simulink model "Periptwsi_2"  (R2020a)
settings: Solver=VariableStepAuto  StartTime=0.0  StopTime=20.0  RelTol=1e-3
undefined symbols (not defined in the file or in its folder): sigbuilder_block
libraries: fuzblock x2
settings Model: Creator=Vasilis Kyrgyrides  LastModifiedBy=Vasilis Kyrgyrides

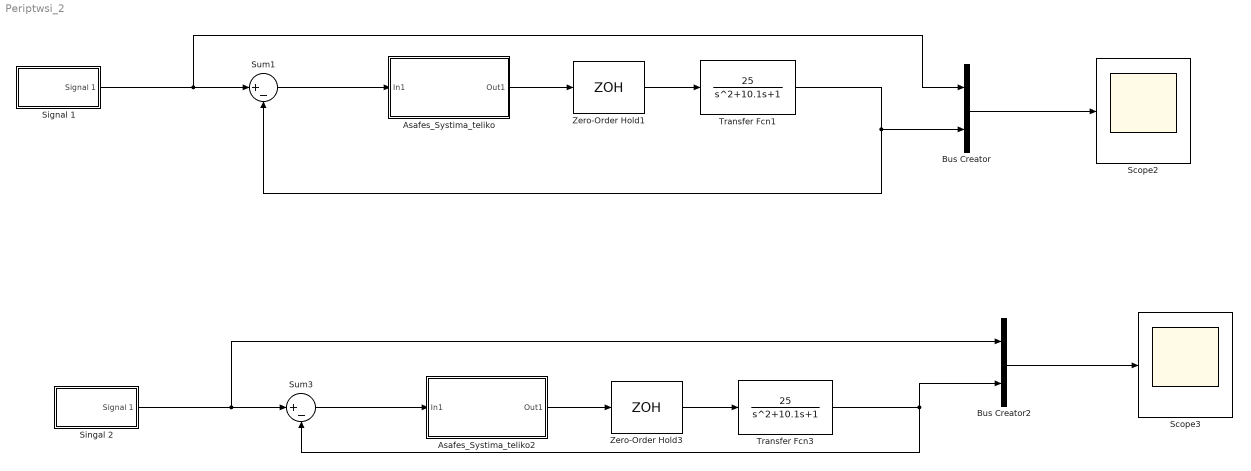
== system Periptwsi_2 ==
  Asafes_Systima_teliko : Subsystem
  Asafes_Systima_teliko2 : Subsystem
  Bus Creator : BusCreator  Inputs=2
  Bus Creator2 : BusCreator  Inputs=2
  Scope2 : Scope
  Scope3 : Scope
  Signal 1 : Subsystem  Tag=STV Subsys  LoadFcn=sigbuilder_block('load');  StartFcn=sigbuilder_block('start');  StopFcn=sigbuilder_block('stop');  ClipboardFcn=sigbuilder_block('clipboard');  mask(Sigbuilder block){tuvar=[0:10]}
      mask help: Simulink:masks:SigbuilderBlock_MD
      mask init:
      | if ~strcmp(get_param(bdroot(gcbh),'SimulationStatus'),'stopped') tuvar = sigbuilder_block('maskInit'); end
      settings: CopyFcn=sigbuilder_block('copy');  DeleteFcn=sigbuilder_block('delete');  ModelCloseFcn=sigbuilder_block('modelClose');  PreSaveFcn=sigbuilder_block('preSave');  PauseFcn=sigbuilder_block('pause');  ContinueFcn=sigbuilder_block('continue');  NameChangeFcn=sigbuilder_block('namechange');  OpenFcn=sigbuilder_block('open',[0.75 30.75 718.5 715.5 ]);  CloseFcn=sigbuilder_block('close');
      mask Display: plot(0, 0, 100, 100,[2, 2, 32, 32, 2], [68, 8, 8, 68, 68],[32, 2], [38, 38], [32, 19, 2],[53, 60, 44], [32, 17, 17, 2],[16, 16, 31, 31]);txt = getActiveGroup(gcbh);text(2, 100, txt,'verticalAlignment', 'top');
  Singal 2 : Subsystem  Tag=STV Subsys  LoadFcn=sigbuilder_block('load');  StartFcn=sigbuilder_block('start');  StopFcn=sigbuilder_block('stop');  ClipboardFcn=sigbuilder_block('clipboard');  mask(Sigbuilder block){tuvar=[0:10]}
      mask help: Simulink:masks:SigbuilderBlock_MD
      mask init:
      | if ~strcmp(get_param(bdroot(gcbh),'SimulationStatus'),'stopped') tuvar = sigbuilder_block('maskInit'); end
      settings: CopyFcn=sigbuilder_block('copy');  DeleteFcn=sigbuilder_block('delete');  ModelCloseFcn=sigbuilder_block('modelClose');  PreSaveFcn=sigbuilder_block('preSave');  PauseFcn=sigbuilder_block('pause');  ContinueFcn=sigbuilder_block('continue');  NameChangeFcn=sigbuilder_block('namechange');  OpenFcn=sigbuilder_block('open',[0.75 30.75 718.5 715.5 ]);  CloseFcn=sigbuilder_block('close');
      mask Display: plot(0, 0, 100, 100,[2, 2, 32, 32, 2], [68, 8, 8, 68, 68],[32, 2], [38, 38], [32, 19, 2],[53, 60, 44], [32, 17, 17, 2],[16, 16, 31, 31]);txt = getActiveGroup(gcbh);text(2, 100, txt,'verticalAlignment', 'top');
  Sum1 : Sum  Inputs=|+-
  Sum3 : Sum  Inputs=|+-
  Transfer Fcn1 : TransferFcn  Numerator=[25]  Denominator=[1 10.1 1]
  Transfer Fcn3 : TransferFcn  Numerator=[25]  Denominator=[1 10.1 1]
  Zero-Order Hold1 : ZeroOrderHold  SampleTime=-1
  Zero-Order Hold3 : ZeroOrderHold  SampleTime=-1
  wires:
  Bus Creator/1 -> Scope2/1
  Sum1/1 -> Asafes_Systima_teliko/1(In1)
  Transfer Fcn1/1 -> Sum1/2, Bus Creator/2
  Signal 1/1(Signal 1) -> Bus Creator/1, Sum1/1
  Zero-Order Hold1/1 -> Transfer Fcn1/1
  Asafes_Systima_teliko/1(Out1) -> Zero-Order Hold1/1
  Zero-Order Hold3/1 -> Transfer Fcn3/1
  Singal 2/1(Signal 1) -> Bus Creator2/1, Sum3/1
  Transfer Fcn3/1 -> Sum3/2, Bus Creator2/2
  Bus Creator2/1 -> Scope3/1
  Sum3/1 -> Asafes_Systima_teliko2/1(In1)
  Asafes_Systima_teliko2/1(Out1) -> Zero-Order Hold3/1

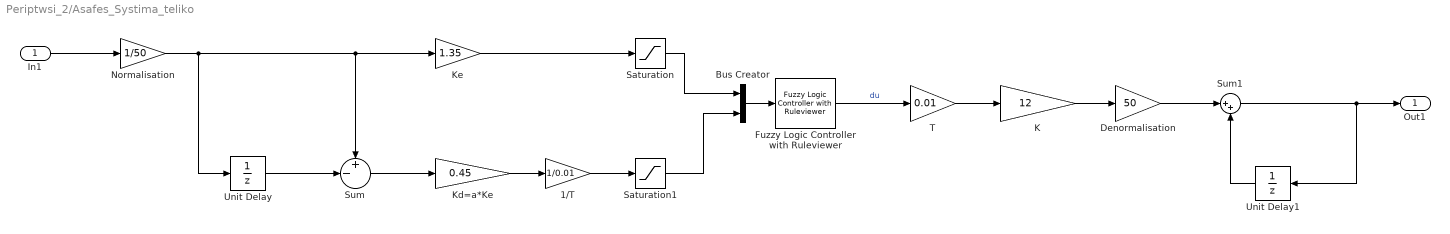
== system Periptwsi_2/Asafes_Systima_teliko ==
  In1 : Inport
  1/T : Gain  Gain=1/0.01
  Bus Creator : BusCreator  Inputs=2
  Denormalisation : Gain  Gain=50
  Fuzzy Logic Controller with Ruleviewer : fuzblock/Fuzzy Logic  Controller  with Ruleviewer  fismatrix=Asafis_PI_2  Ts=0.01
  K : Gain  Gain=12
  Kd=a*Ke : Gain  Gain=0.45
  Ke : Gain  Gain=1.35
  Normalisation : Gain  Gain=1/50
  Saturation : Saturate  UpperLimit=1  LowerLimit=-1
  Saturation1 : Saturate  UpperLimit=1  LowerLimit=-1
  Sum : Sum  Inputs=+-|
  Sum1 : Sum  Inputs=|++
  T : Gain  Gain=0.01
  Unit Delay : UnitDelay  SampleTime=-1  HasFrameUpgradeWarning=on
  Unit Delay1 : UnitDelay  SampleTime=-1  HasFrameUpgradeWarning=on
  Out1 : Outport
  wires:
  In1/1 -> Normalisation/1
  Unit Delay/1 -> Sum/2
  Normalisation/1 -> Sum/1, Ke/1, Unit Delay/1
  Sum/1 -> Kd=a*Ke/1
  Kd=a*Ke/1 -> 1/T/1
  Ke/1 -> Saturation/1
  1/T/1 -> Saturation1/1
  Saturation1/1 -> Bus Creator/2
  Saturation/1 -> Bus Creator/1
  K/1 -> Denormalisation/1
  T/1 -> K/1
  Fuzzy Logic Controller with Ruleviewer/1 -> T/1  "du"
  Denormalisation/1 -> Sum1/1
  Sum1/1 -> Unit Delay1/1, Out1/1
  Unit Delay1/1 -> Sum1/2
  Bus Creator/1 -> Fuzzy Logic Controller with Ruleviewer/1

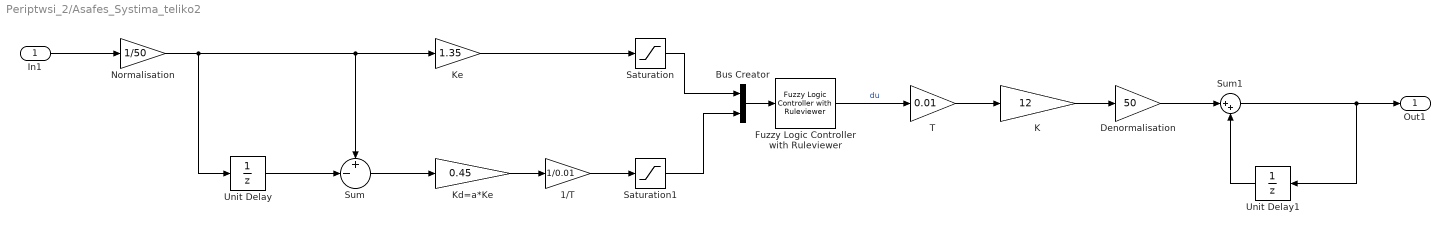
== system Periptwsi_2/Asafes_Systima_teliko2 ==
  In1 : Inport
  1/T : Gain  Gain=1/0.01
  Bus Creator : BusCreator  Inputs=2
  Denormalisation : Gain  Gain=50
  Fuzzy Logic Controller with Ruleviewer : fuzblock/Fuzzy Logic  Controller  with Ruleviewer  fismatrix=Asafis_PI_2  Ts=0.01
  K : Gain  Gain=12
  Kd=a*Ke : Gain  Gain=0.45
  Ke : Gain  Gain=1.35
  Normalisation : Gain  Gain=1/50
  Saturation : Saturate  UpperLimit=1  LowerLimit=-1
  Saturation1 : Saturate  UpperLimit=1  LowerLimit=-1
  Sum : Sum  Inputs=+-|
  Sum1 : Sum  Inputs=|++
  T : Gain  Gain=0.01
  Unit Delay : UnitDelay  SampleTime=-1  HasFrameUpgradeWarning=on
  Unit Delay1 : UnitDelay  SampleTime=-1  HasFrameUpgradeWarning=on
  Out1 : Outport
  wires:
  In1/1 -> Normalisation/1
  Unit Delay/1 -> Sum/2
  Normalisation/1 -> Sum/1, Ke/1, Unit Delay/1
  Sum/1 -> Kd=a*Ke/1
  Kd=a*Ke/1 -> 1/T/1
  Ke/1 -> Saturation/1
  1/T/1 -> Saturation1/1
  Saturation1/1 -> Bus Creator/2
  Saturation/1 -> Bus Creator/1
  K/1 -> Denormalisation/1
  T/1 -> K/1
  Fuzzy Logic Controller with Ruleviewer/1 -> T/1  "du"
  Denormalisation/1 -> Sum1/1
  Sum1/1 -> Unit Delay1/1, Out1/1
  Unit Delay1/1 -> Sum1/2
  Bus Creator/1 -> Fuzzy Logic Controller with Ruleviewer/1

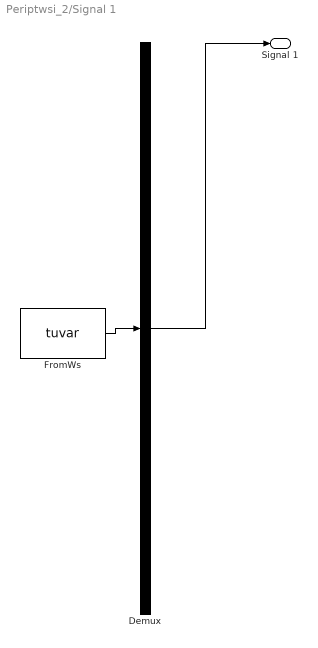
== system Periptwsi_2/Signal 1 ==
  Demux : Demux  Tag=STV Demux  Outputs=1
      settings: DisplayOption=none
  FromWs : FromWorkspace  Tag=STV FromWs  VariableName=tuvar
      SigBuilderData=|
      | common.afterFinalStr = 'Extrapolate'
      | common.sampleTime = 0
      | dataSet.timeRange = [0 20]
      | dataSet.name = 'Pulse'
      | sbobj.Groups.Name = 'Pulse'
      | sbobj.Groups.Signals.Name = 'Signal 1'
      | sbobj.Groups.Signals.XData = [0 5 5 10 10 20]
      | sbobj.Groups.Signals.YData = [50 50 20 20 40 40]
      | sbobj.Groups.TimeRange = [0 20]
  Signal 1 : Outport  Tag=STV Outport  VectorParamsAs1DForOutWhenUnconnected=off
  wires:
  Demux/1 -> Signal 1/1
  FromWs/1 -> Demux/1

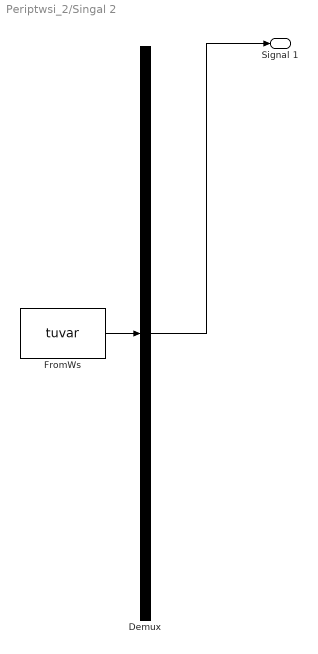
== system Periptwsi_2/Singal 2 ==
  Demux : Demux  Tag=STV Demux  Outputs=1
      settings: DisplayOption=none
  FromWs : FromWorkspace  Tag=STV FromWs  VariableName=tuvar
      SigBuilderData=|
      | common.afterFinalStr = 'Extrapolate'
      | common.sampleTime = 0
      | dataSet.timeRange = [0 20]
      | dataSet.name = 'Trapezodial'
      | sbobj.Groups.Name = 'Trapezodial'
      | sbobj.Groups.Signals.Name = 'Signal 1'
      | sbobj.Groups.Signals.XData = [0 5 10 16 20]
      | sbobj.Groups.Signals.YData = [0 50 49.8 20 0]
      | sbobj.Groups.TimeRange = [0 20]
  Signal 1 : Outport  Tag=STV Outport  VectorParamsAs1DForOutWhenUnconnected=off
  wires:
  Demux/1 -> Signal 1/1
  FromWs/1 -> Demux/1
